simulink model "sim_model_dynamic"  (R2015a)
settings: Solver=ode45  StartTime=0.0  StopTime=11  RelTol=1e-12
undefined symbols (not defined in the file or in its folder): a1, a2, b1, c1, Cyf, Cyr, Cyt, e1, Iz1, Iz2, L, L1, L12, L2, l2, m1, m2, v, vx
settings Model: Creator=Luis F  LastModifiedBy=Luis F

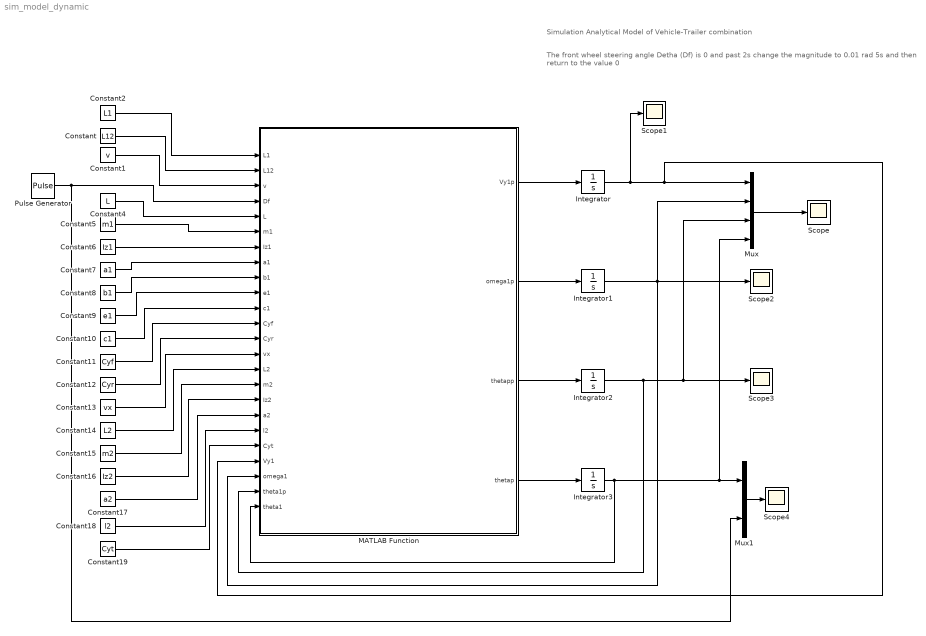
== system sim_model_dynamic ==
  note: Simulation Analytical Model of Vehicle-Trailer combination
  note: The front wheel steering angle Detha (Df) is 0 and past 2s change the magnitude to 0.01 rad 5s and then return to the value 0
  Constant : Constant  Value=L12
  Constant1 : Constant  Value=v
  Constant10 : Constant  Value=c1
  Constant11 : Constant  Value=Cyf
  Constant12 : Constant  Value=Cyr
  Constant13 : Constant  Value=vx
  Constant14 : Constant  Value=L2
  Constant15 : Constant  Value=m2
  Constant16 : Constant  Value=Iz2
  Constant17 : Constant  Value=a2
  Constant18 : Constant  Value=l2
  Constant19 : Constant  Value=Cyt
  Constant2 : Constant  Value=L1
  Constant4 : Constant  Value=L
  Constant5 : Constant  Value=m1
  Constant6 : Constant  Value=Iz1
  Constant7 : Constant  Value=a1
  Constant8 : Constant  Value=b1
  Constant9 : Constant  Value=e1
  Integrator{,1..3} (4 alike) : Integrator
  MATLAB Function : MATLAB Function  TreatAsAtomicUnit=on
  Mux : Mux
  Mux1 : Mux  Inputs=2
  Pulse Generator : DiscretePulseGenerator  PulseType=Time based  Amplitude=0.001  Period=10  PulseWidth=50  PhaseDelay=2
  Scope{,1..4} (5 alike) : Scope
      Scope2 settings: SaveName=ScopeData2
      Scope3 settings: SaveName=ScopeData3
      Scope4 settings: SaveName=ScopeData4
  wires:
  Constant2/1 -> MATLAB Function/1(L1)
  Constant/1 -> MATLAB Function/2(L12)
  Constant1/1 -> MATLAB Function/3(v)
  Pulse Generator/1 -> Mux1/2, MATLAB Function/4(Df)
  Constant4/1 -> MATLAB Function/5(L)
  Constant5/1 -> MATLAB Function/6(m1)
  Constant6/1 -> MATLAB Function/7(Iz1)
  Constant7/1 -> MATLAB Function/8(a1)
  Constant8/1 -> MATLAB Function/9(b1)
  Constant9/1 -> MATLAB Function/10(e1)
  Constant10/1 -> MATLAB Function/11(c1)
  Constant11/1 -> MATLAB Function/12(Cyf)
  Constant12/1 -> MATLAB Function/13(Cyr)
  Constant13/1 -> MATLAB Function/14(vx)
  Constant14/1 -> MATLAB Function/15(L2)
  Constant15/1 -> MATLAB Function/16(m2)
  Constant16/1 -> MATLAB Function/17(Iz2)
  Constant17/1 -> MATLAB Function/18(a2)
  Constant18/1 -> MATLAB Function/19(l2)
  Constant19/1 -> MATLAB Function/20(Cyt)
  MATLAB Function/4(thetap) -> Integrator3/1
  MATLAB Function/3(thetapp) -> Integrator2/1
  MATLAB Function/2(omega1p) -> Integrator1/1
  MATLAB Function/1(Vy1p) -> Integrator/1
  Integrator1/1 -> Scope2/1, Mux/2, MATLAB Function/22(omega1)
  Integrator3/1 -> MATLAB Function/24(theta1), Mux/4, Mux1/1
  Integrator2/1 -> MATLAB Function/23(theta1p), Scope3/1, Mux/3
  Mux/1 -> Scope/1
  Integrator/1 -> Scope1/1, MATLAB Function/21(Vy1), Mux/1
  Mux1/1 -> Scope4/1

== matlab function sim_model_dynamic/MATLAB Function ==
  data: L1 input; Vy1p output; L12 input; v input; Df input; L input; m1 input; Iz1 input; a1 input; b1 input; e1 input; c1 input; Cyf input; Cyr input; vx input; L2 input; m2 input; Iz2 input; a2 input; l2 input; Cyt input; Vy1 input; omega1 input; theta1p input; theta1 input; omega1p output; thetapp output; thetap output
function [Vy1p, omega1p, thetapp, thetap]  = fcn(L1,L12,v,Df,L,m1,Iz1,a1,b1,e1,c1,Cyf,Cyr,vx,L2,m2,Iz2,a2,l2,Cyt,Vy1,omega1,theta1p,theta1)


    M =[m1+m2,-m2*(c1+a2),-m2*a2,0;
       m1*c1,Iz1,0,0;
       -m2*a2,Iz2+(m2*a2*(c1+a2)),Iz2+(m2*a2^2),0;
       0,0,0,1];
 
    D =[-(Cyf+Cyr+Cyt)/vx,((-Cyf*a1)+(Cyr*b1)+(Cyt*(c1+12))-((m1+m2)*vx^2))/vx,Cyt*l2/vx,Cyt;
       -(Cyf*(a1+c1)+Cyr*e1)/vx, (-Cyf*a1*(a1+c1)+(Cyr*b1*e1)-(m1*c1*vx^2))/vx, 0, 0;
       (Cyt*l2)/vx,-(Cyt*l2*(c1+l2)+m2*a2*vx^2)/vx,-(Cyt*l2^2)/vx,-Cyt*l2;
       0,0,1,0];
   
    E=[Cyf, 0, 0;
       Cyf*(a1+c1), 1, 0;
       0, 0, 1;
       0, 0, 0];

    F=[1 1;
      c1, 0;
      0, -a2;
      0, 0];

    A=inv(M)*D;
    B=inv(M)*E;
    G=inv(M)*F;
    
    u=(Df-theta1)*Iz1;
    
    Vy1p=(A(1,1)*Vy1)+(A(1,2)*omega1)+(A(1,3)*theta1p)+(A(1,4)*theta1)+(B(1,1)+B(1,2)+B(1,3))*u+(G(1,1)+G(1,2))*Df;
    omega1p=(A(2,1)*Vy1)+(A(2,2)*omega1)+(A(2,3)*theta1p)+(A(2,4)*theta1)+(B(2,1)+B(2,2)+B(2,3))*u+(G(2,1)+G(2,2))*Df;
    thetapp=(A(3,1)*Vy1)+(A(3,2)*omega1)+(A(3,3)*theta1p)+(A(3,4)*theta1)+(B(3,1)+B(3,2)+B(3,3))*u+(G(3,1)+G(3,2))*Df;
    thetap=(A(4,1)*Vy1)+(A(4,2)*omega1)+(A(4,3)*theta1p)+(A(4,4)*theta1)+(B(4,1)+B(4,2)+B(4,3))*u+(G(4,1)+G(4,2))*Df;
